simulink model "mavsim_chap4_R2016b"  (R2016b)
settings: Solver=ode45  StartTime=0.0  StopTime=10000  RelTol=1e-3  EnableMultiTasking=on
InitFcn:
  | Params
values from neighbouring files (symbols this model uses):
  P = load('aerosonde_data.mat')    [Params.m]
undefined symbols (not defined in the file or in its folder): airdata, drawAircraft, forces_moments, plotMAVStateVariables
libraries: simulink x4
settings Model: Creator=beard  LastModifiedBy=João Pinto
settings DataIOCC: LimitDataPoints=on  SaveFormat=Array  SignalLoggingSaveFormat=ModelDataLogs
settings OptimizationCC: ExpressionDepthLimit=2147483647  InitFltsAndDblsToZero=on  LifeSpan=inf
settings DebuggingCC: UnderspecifiedInitializationDetection=Classic  MergeDetectMultiDrivingBlocksExec=none  SolverPrmCheckMsg=warning  FcnCallInpInsideContextMsg=warning  StateNameClashWarn=warning  SFUnexpectedBacktrackingDiag=warning  SFNoUnconditionalDefaultTransitionDiag=warning  SFExecutionAtInitializationDiag=none
settings HardwareCC: ProdBitPerPointer=32  ProdBitPerSizeT=32  ProdBitPerPtrDiffT=32  ProdLargestAtomicFloat=None  ProdIntDivRoundTo=Undefined  ProdEndianess=Unspecified  ProdWordSize=32  ProdHWDeviceType=32-bit Generic
settings ModelReferenceCC: PropagateSignalLabelsOutOfModel=off
settings GRTTargetCC: TargetLangStandard=C89/C90 (ANSI)  GeneratePreprocessorConditionals=Disable all  CombineOutputUpdateFcns=off  GRTInterface=on
settings ConfigComp: CovMetricSettings=dw  CovHtmlReporting=on  CovSaveCumulativeToWorkspaceVar=on  CovSaveSingleToWorkspaceVar=on  CovExternalEMLEnable=off  CovSFcnEnable=off

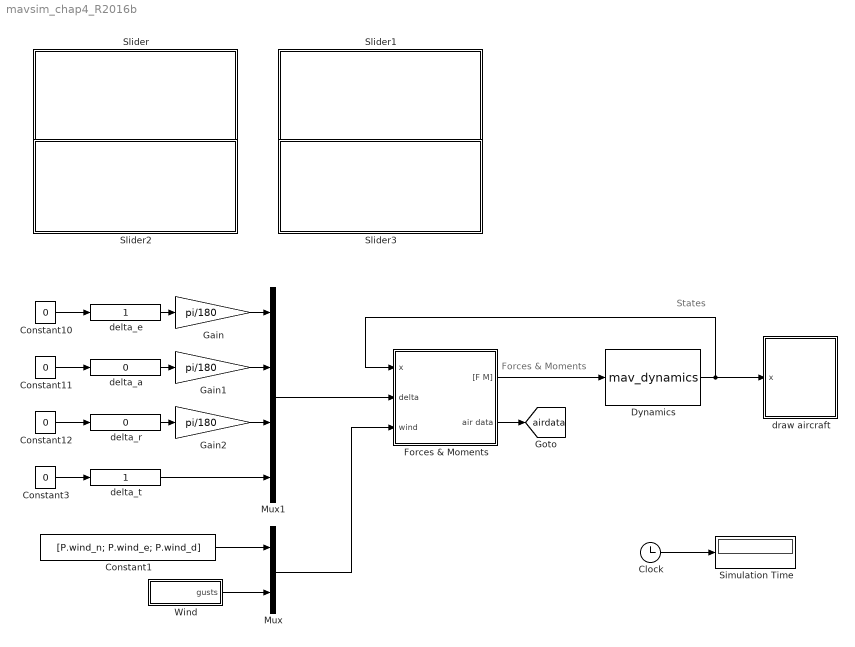
== system mavsim_chap4_R2016b ==
  note: Forces & Moments
  note: States
  Clock : Clock
  Constant1 : Constant  Value=[P.wind_n; P.wind_e; P.wind_d]
  Constant{3,10..12} (4 alike) : Constant  Value=0
  Dynamics : S-Function  FunctionName=mav_dynamics  Parameters=P  SFunctionDeploymentMode=off  EnableBusSupport=off
  Forces & Moments : Subsystem
  Gain : Gain  Gain=pi/180
  Gain1 : Gain  Gain=pi/180
  Gain2 : Gain  Gain=pi/180
  Mux : Mux  Inputs=2
  Mux1 : Mux
  Simulation Time : Display
  Slider : Subsystem  DialogController=hmiCreateDDGDialog  IsWebBlock=on  mask(MWDashboardBlock){webBlockId=eb490caa-51d8-4fad-a98f-bb1481b8ab94, webBlockType=slider, ShowInLibBrowser=on, ShowInitialText=on, HMISrcModelName=mavsim_chap4_R2016b}
      mask prompts: webBlockId "WebBlock Id"; webBlockType "WebBlock Type"; HMISrcModelName "Source Model"
      mask help: SimulinkHMI:dialogs:SliderDialogDesc
      mask Help: helpview([docroot '/mapfiles/simulink.map'], 'hmi_slider')
      mask Display:
      | if strcmp(get_param(bdroot(gcb),'BlockDiagramType'), 'library')
      |     image([(matlabroot) '/toolbox/simulink/hmi/icons/Slider.png']);
      | end
  Slider1 : Subsystem  DialogController=hmiCreateDDGDialog  IsWebBlock=on  mask(MWDashboardBlock){webBlockId=f2585cef-4bce-46a0-b255-849fc52a219f, webBlockType=slider, ShowInLibBrowser=on, ShowInitialText=on, HMISrcModelName=mavsim_chap4_R2016b}
      mask prompts: webBlockId "WebBlock Id"; webBlockType "WebBlock Type"; HMISrcModelName "Source Model"
      mask help: SimulinkHMI:dialogs:SliderDialogDesc
      mask Help: helpview([docroot '/mapfiles/simulink.map'], 'hmi_slider')
      mask Display:
      | if strcmp(get_param(bdroot(gcb),'BlockDiagramType'), 'library')
      |     image([(matlabroot) '/toolbox/simulink/hmi/icons/Slider.png']);
      | end
  Slider2 : Subsystem  DialogController=hmiCreateDDGDialog  IsWebBlock=on  mask(MWDashboardBlock){webBlockId=8c9d0b31-bde6-497a-8c29-d58406641278, webBlockType=slider, ShowInLibBrowser=on, ShowInitialText=on, HMISrcModelName=mavsim_chap4_R2016b}
      mask prompts: webBlockId "WebBlock Id"; webBlockType "WebBlock Type"; HMISrcModelName "Source Model"
      mask help: SimulinkHMI:dialogs:SliderDialogDesc
      mask Help: helpview([docroot '/mapfiles/simulink.map'], 'hmi_slider')
      mask Display:
      | if strcmp(get_param(bdroot(gcb),'BlockDiagramType'), 'library')
      |     image([(matlabroot) '/toolbox/simulink/hmi/icons/Slider.png']);
      | end
  Slider3 : Subsystem  DialogController=hmiCreateDDGDialog  IsWebBlock=on  mask(MWDashboardBlock){webBlockId=efb7b97b-68c6-4dfd-8944-a26475207f22, webBlockType=slider, ShowInLibBrowser=on, ShowInitialText=on, HMISrcModelName=mavsim_chap4_R2016b}
      mask prompts: webBlockId "WebBlock Id"; webBlockType "WebBlock Type"; HMISrcModelName "Source Model"
      mask help: SimulinkHMI:dialogs:SliderDialogDesc
      mask Help: helpview([docroot '/mapfiles/simulink.map'], 'hmi_slider')
      mask Display:
      | if strcmp(get_param(bdroot(gcb),'BlockDiagramType'), 'library')
      |     image([(matlabroot) '/toolbox/simulink/hmi/icons/Slider.png']);
      | end
  Wind : Subsystem
  delta_a : simulink/Math Operations/Slider Gain  gain=0  low=-45  high=45
  delta_e : simulink/Math Operations/Slider Gain  gain=1  low=-45  high=45
  delta_r : simulink/Math Operations/Slider Gain  gain=0  low=-45  high=45
  delta_t : simulink/Math Operations/Slider Gain  gain=1  low=0  high=1
  draw aircraft : Subsystem
      mask Display: image(imread('tv.jpg'))
  tag scope: airdata=global
  wires:
  Constant10/1 -> delta_e/1
  Constant11/1 -> delta_a/1
  Constant12/1 -> delta_r/1
  Dynamics/1 -> draw aircraft/1(x), Forces & Moments/1(x)
  delta_r/1 -> Gain2/1
  delta_a/1 -> Gain1/1
  delta_e/1 -> Gain/1
  Constant3/1 -> delta_t/1
  delta_t/1 -> Mux1/4
  Mux1/1 -> Forces & Moments/2(delta)
  Forces & Moments/1("[F M]") -> Dynamics/1
  Clock/1 -> Simulation Time/1
  Mux/1 -> Forces & Moments/3(wind)
  Constant1/1 -> Mux/1
  Forces & Moments/2(air data) -> [airdata]
  Gain/1 -> Mux1/1
  Gain1/1 -> Mux1/2
  Gain2/1 -> Mux1/3
  Wind/1(gusts) -> Mux/2

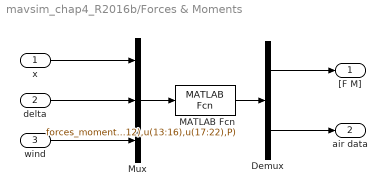
== system mavsim_chap4_R2016b/Forces & Moments ==
  x : Inport
  delta : Inport  Port=2
  wind : Inport  Port=3
  Demux : Demux  Outputs=[6;6]
  MATLAB Fcn : MATLABFcn  MATLABFcn=forces_moments(u(1:12),u(13:16),u(17:22),P)  OutputDimensions=12
  Mux : Mux  Inputs=3
  "[F M]" : Outport
  air data : Outport  Port=2
  wires:
  x/1 -> Mux/1
  delta/1 -> Mux/2
  wind/1 -> Mux/3
  MATLAB Fcn/1 -> Demux/1
  Demux/1 -> "[F M]"/1
  Mux/1 -> MATLAB Fcn/1
  Demux/2 -> air data/1

== system mavsim_chap4_R2016b/Slider ==

== system mavsim_chap4_R2016b/Slider1 ==

== system mavsim_chap4_R2016b/Slider2 ==

== system mavsim_chap4_R2016b/Slider3 ==

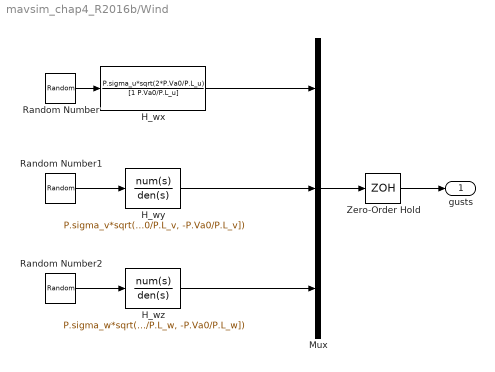
== system mavsim_chap4_R2016b/Wind ==
  H_wx : TransferFcn  Numerator=P.sigma_u*sqrt(2*P.Va0/P.L_u)  Denominator=[1 P.Va0/P.L_u]
  H_wy : TransferFcn  Numerator=P.sigma_v*sqrt(3*P.Va0/P.L_v)*[0, 1, P.Va0/sqrt(3)/P.L_v]  Denominator=poly([-P.Va0/P.L_v, -P.Va0/P.L_v])
  H_wz : TransferFcn  Numerator=P.sigma_w*sqrt(3*P.Va0/P.L_w)*[0, 1, P.Va0/sqrt(3)/P.L_w]  Denominator=poly([-P.Va0/P.L_w, -P.Va0/P.L_w])
  Mux : Mux  Inputs=3
  Random Number : RandomNumber  SampleTime=0
  Random Number1 : RandomNumber  SampleTime=0
  Random Number2 : RandomNumber  SampleTime=0
  Zero-Order Hold : ZeroOrderHold  SampleTime=P.Ts
  gusts : Outport
  wires:
  H_wx/1 -> Mux/1
  Random Number/1 -> H_wx/1
  H_wy/1 -> Mux/2
  Random Number1/1 -> H_wy/1
  H_wz/1 -> Mux/3
  Random Number2/1 -> H_wz/1
  Mux/1 -> Zero-Order Hold/1
  Zero-Order Hold/1 -> gusts/1

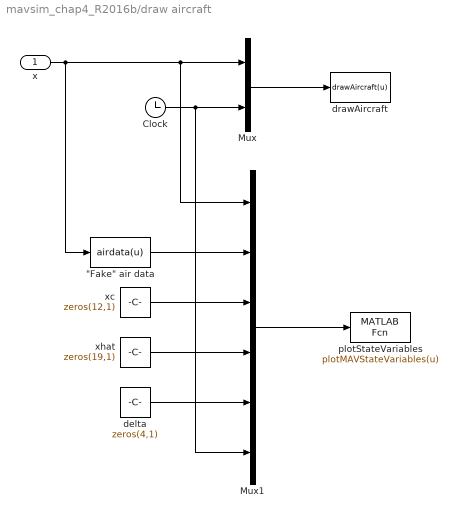
== system mavsim_chap4_R2016b/draw aircraft ==
  x : Inport
  "\"Fake\" air data" : MATLABFcn  MATLABFcn=airdata(u)  OutputDimensions=6  SampleTime=0.1
  Clock : Clock
  Mux : Mux  Inputs=2
  Mux1 : Mux  Inputs=6
  delta : Constant  Value=zeros(4,1)
  drawAircraft : MATLABFcn  MATLABFcn=drawAircraft(u)  OutputDimensions=0  SampleTime=0.1
  plotStateVariables : MATLABFcn  MATLABFcn=plotMAVStateVariables(u)  OutputDimensions=0  SampleTime=0.1
  xc : Constant  Value=zeros(12,1)
  xhat : Constant  Value=zeros(19,1)
  wires:
  "\"Fake\" air data"/1 -> Mux1/2
  delta/1 -> Mux1/5
  xc/1 -> Mux1/3
  xhat/1 -> Mux1/4
  Mux1/1 -> plotStateVariables/1
  Clock/1 -> Mux1/6, Mux/2
  x/1 -> "\"Fake\" air data"/1, Mux1/1, Mux/1
  Mux/1 -> drawAircraft/1
